simulink model "TDM_P3_v2006b"  (Simulink 6.5)
settings: Solver=ode45  StartTime=0.0  StopTime=10.0  RelTol=1e-3
libraries: simeventsattributes1 x3, simeventsgenerators1 x3, simeventssink1 x2, simeventsrouting1 x1, simulink x1
settings Model: Creator=mclune  LastModifiedBy=generica  ExtModeAutoUpdateStatusClock=off
settings DebuggingCC: SolverPrmCheckMsg=none  MultiTaskDSMMsg=warning  MultiTaskCondExecSysMsg=none  SigSpecEnsureSampleTimeMsg=none  StrictBusMsg=None
settings RTWCC: IncludeERTFirstTime=on
settings SimEventsCC: propIdentEventSeed=12345678  propLogEventsScheduled=0  propLogEventsExecuted=0  propLogDepartureEvents=0  propDisplayEventCalendar=0

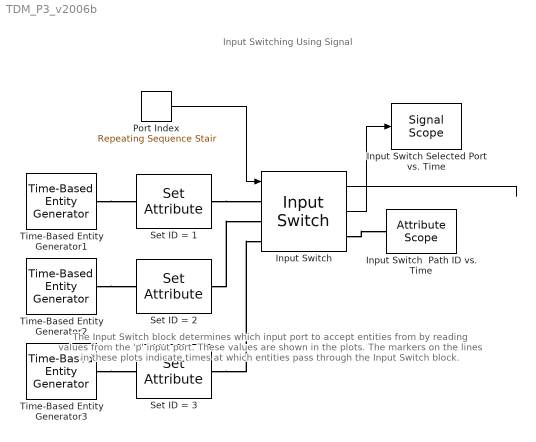
== system TDM_P3_v2006b ==
  note: Input Switching Using Signal
  note: The Input Switch block determines which input port to
      | accept entities from by reading values from the 'p'
      | input port.  These values are shown in the plots.  The
      | markers on the lines in these plots indicate times at
      | which entities pass through the Input Switch block.
  Input Switch : simeventsrouting1/Input Switch  Priority=1  SystemSampleTime=-1  NumberInputPorts=3  SwitchingCriterion=From signal port p  InitialSeed=23456  SpecifyEventPriority=on  PriorityInputSwitchSelectPort=1  StatNumberDeparted=On  StatLastArrivalPort=On
  Input Switch Selected Port vs. Time : simeventssink1/Signal Scope  Priority=1  SystemSampleTime=-1  PlotType=Stair  InputType=Signal  NumInputs=1  AttributeNameY=Count  XInputOptionSignal=Event time  XInputOptionEntity=Event time  AttributeNameX=Count  EnableEntityOutport=on  XMin=0  XMax=10  XLimitExceededOption=Stretch axis limits  YLimitExceededOption=Stretch axis limits  AxisGrid=on  AxisLegend=off  LineDisables=""  LineColors=b  LineStyles=-  LineMarkers=.  OpenScopeAtSimStart=on  Title=Selected Port vs. Time  YLabel=Selected Port  XLabel=Time  FigurePosition=[603 400 350 262]  AxisZoom=off  DataStoreOption=Limited  DataPointsLimit=10000  StatNumberArrived=Off  ShowCountPlotted=off  ShowToolbar=on
      settings: YMin=0  YMax=4
  Input Switch  Path ID vs. Time : simeventssink1/Attribute Scope  Priority=1  SystemSampleTime=-1  PlotType=Stair  InputType=Attribute  NumInputs=1  AttributeNameY=ID  XInputOptionSignal=Event time  XInputOptionEntity=Event time  AttributeNameX=Count  EnableEntityOutport=off  XMin=0  XMax=10  XLimitExceededOption=Stretch axis limits  YLimitExceededOption=Stretch axis limits  AxisGrid=on  AxisLegend=off  LineDisables=""  LineColors=b  LineStyles=-  LineMarkers=.  OpenScopeAtSimStart=on  Title=Entity Path ID vs. Time  YLabel=Path ID  XLabel=Time  FigurePosition=[603 50 350 263]  AxisZoom=off  DataStoreOption=Limited  DataPointsLimit=10000  StatNumberArrived=Off  ShowCountPlotted=off  ShowToolbar=on
      settings: YMin=0  YMax=4
  Port Index : simulink/Sources/Repeating Sequence Stair  SystemSampleTime=-1  OutValues=[1 2 3].'  tsamp=1  OutputDataTypeScalingMode=Specify via dialog  OutDataType=float('double')  ConRadixGroup=Best Precision: Vector-wise  OutScaling=2^-12
      settings: AttributesFormatString=Sequence = %<OutValues>\nSample Time: %<tsamp>
  Set ID = 1 : simeventsattributes1/Set Attribute  Priority=1  SystemSampleTime=-1  Attribute1From=Specify via dialog  Attribute1Name=ID  Attribute1DataType=Double  Attribute1Value=1  Attribute1Create=on  Attribute2From=Off  Attribute2Name=Attribute2  Attribute2DataType=Double  Attribute2Value=0  Attribute2Create=on  Attribute3From=Off  Attribute3Name=Attribute3  Attribute3DataType=Double  Attribute3Value=0  Attribute3Create=on  Attribute4From=Off  Attribute4Name=Attribute4  Attribute4DataType=Double  Attribute4Value=0  Attribute4Create=on  StatNumberDeparted=Off
  Set ID = 2 : simeventsattributes1/Set Attribute  Priority=1  SystemSampleTime=-1  Attribute1From=Specify via dialog  Attribute1Name=ID  Attribute1DataType=Double  Attribute1Value=2  Attribute1Create=on  Attribute2From=Off  Attribute2Name=Attribute2  Attribute2DataType=Double  Attribute2Value=0  Attribute2Create=on  Attribute3From=Off  Attribute3Name=Attribute3  Attribute3DataType=Double  Attribute3Value=0  Attribute3Create=on  Attribute4From=Off  Attribute4Name=Attribute4  Attribute4DataType=Double  Attribute4Value=0  Attribute4Create=on  StatNumberDeparted=Off
  Set ID = 3 : simeventsattributes1/Set Attribute  Priority=1  SystemSampleTime=-1  Attribute1From=Specify via dialog  Attribute1Name=ID  Attribute1DataType=Double  Attribute1Value=3  Attribute1Create=on  Attribute2From=Off  Attribute2Name=Attribute2  Attribute2DataType=Double  Attribute2Value=0  Attribute2Create=on  Attribute3From=Off  Attribute3Name=Attribute3  Attribute3DataType=Double  Attribute3Value=0  Attribute3Create=on  Attribute4From=Off  Attribute4Name=Attribute4  Attribute4DataType=Double  Attribute4Value=0  Attribute4Create=on  StatNumberDeparted=Off
  Time-Based Entity Generator1 : simeventsgenerators1/Entity Generators/Time-Based Entity Generator  Priority=1  DialogController=des_ddg_create  DialogControllerArgs=DataTag7  SystemSampleTime=-1  GenerateEntitiesUpon=Intergeneration time from dialog  Distribution=Constant  Minimum=0  Maximum=1  Mean=1  InitialSeed=12345  Period=.01  PriorityEntityGeneration=2  GenerateEntityAtSimulationStart=on  ResponseWhenBlocked=Pause generation  ResponseWhenUnblocked=Immediate restart  EntityType=Standard  StatNumberDeparted=Off  StatPendingEntity=Off  StatAverageIntergenerationTime=Off
  Time-Based Entity Generator2 : simeventsgenerators1/Entity Generators/Time-Based Entity Generator  Priority=1  DialogController=des_ddg_create  DialogControllerArgs=DataTag9  SystemSampleTime=-1  GenerateEntitiesUpon=Intergeneration time from dialog  Distribution=Constant  Minimum=0  Maximum=1  Mean=1  InitialSeed=12345  Period=0.30  PriorityEntityGeneration=3  GenerateEntityAtSimulationStart=on  ResponseWhenBlocked=Pause generation  ResponseWhenUnblocked=Immediate restart  EntityType=Standard  StatNumberDeparted=Off  StatPendingEntity=Off  StatAverageIntergenerationTime=Off
  Time-Based Entity Generator3 : simeventsgenerators1/Entity Generators/Time-Based Entity Generator  Priority=1  DialogController=des_ddg_create  DialogControllerArgs=DataTag11  SystemSampleTime=-1  GenerateEntitiesUpon=Intergeneration time from dialog  Distribution=Constant  Minimum=0  Maximum=1  Mean=1  InitialSeed=12345  Period=1  PriorityEntityGeneration=2  GenerateEntityAtSimulationStart=on  ResponseWhenBlocked=Pause generation  ResponseWhenUnblocked=Immediate restart  EntityType=Standard  StatNumberDeparted=Off  StatPendingEntity=Off  StatAverageIntergenerationTime=Off
  wires:
  Input Switch/2 -> Input Switch Selected Port vs. Time/1
  Port Index/1 -> Input Switch/1
  Input Switch/1 -> ?
  connections:
  Set ID = 1/RConn1 -- Input Switch/LConn1
  Set ID = 2/RConn1 -- Input Switch/LConn2
  Input Switch/RConn1 -- Input Switch  Path ID vs. Time/LConn1
  Time-Based Entity Generator1/RConn1 -- Set ID = 1/LConn1
  Time-Based Entity Generator2/RConn1 -- Set ID = 2/LConn1
  Set ID = 3/RConn1 -- Input Switch/LConn3
  Time-Based Entity Generator3/RConn1 -- Set ID = 3/LConn1
